simulink model "Mpc_SimMechanics_with_standing"  (R2017b)
settings: Solver=ode45  StartTime=0  StopTime=10  FixedStep=0.0005  EnableMultiTasking=on
InitFcn:
  | isSim = 1;
  | 
  | PreFunctions.CustomInitFcn_with_standing;
  | PreFunctions.simulationInitFcn_with_standing;
undefined symbols (not defined in the file): alpha_x, alpha_y, DiagnosticCodes, DynamicMatrixLibrary, motorPositions, motorVelocities, pelvisPosition, pelvisVelocity, sample_time, X, Y, Z
libraries: sm_lib x170, nesl_utility x75, Contact_Forces_Lib x6, ComponentLibrary x5, xpcrtudplib x2, slrtlib x1
(part 4 of 8)

== system Mpc_SimMechanics_with_standing/Cassie/Cassie Simulation/Cassie Pelvis ==
  Bus Element In : Inport  PortName=InBus  Element=radio
  Battery : ComponentLibrary/Simulation/Battery  SystemSampleTime=-1
  Pelvis Solid : sm_lib/Body Elements/Solid  InertiaType=Custom  Mass=10.33  MassUnits=kg  CenterOfMass=[0.05066 0.000346 0.02841]  CenterOfMassUnits=m  MomentsOfInertia=[0.085821 0.049222 0.08626]  MomentsOfInertiaUnits=kg*m^2  ProductsOfInertia=[1.276e-05 -0.00016022 -0.000414]  ProductsOfInertiaUnits=kg*m^2  DensityBased=on  Density=1000  DensityUnits=kg/(m^3)  DoExposeReferenceFrame=on  SerializedFrames=<Frames/>  GraphicType=FromGeometry  MarkerShape=Sphere  MarkerSize=10  GraphicVisPropType=SimpleVisualProperties  GraphicDiffuseColor=[0.8 0.8 0.8]  GraphicSpecularColor=[0.5 0.5 0.5 1.0]  GraphicAmbientColor=[0.5 0.5 0.5 1.0]  GraphicEmissiveColor=[0.5 0.5 0.5 1.0]  GraphicShininess=75  GraphicOpacity=1.0  GeometryShape=FromFile  RectangleSize=[1 1]  RectangleSizeUnits=m  BrickDimensions=[1 1 1]  BrickDimensionUnits=m  CylinderRadius=1  CylinderRadiusUnits=m  CylinderLength=1  CylinderLengthUnits=m  SphereRadius=1  SphereRadiusUnits=m  EllipsoidRadii=[1 1 1]  EllipsoidRadiiUnits=m  ExtrusionCrossSection=[1 1; -1 1; -1 -1; 1 -1]  ExtrusionCrossSectionUnits=m  ExtrusionLength=1  ExtrusionLengthUnits=m  PolygonNumSides=3  PolygonOuterRadius=1  PolygonOuterRadiusUnits=m  ExtGeomFileType=STL  ExtGeomFileName=cassie-pelvis.stl  ExtGeomFileUnits=m  RevolutionCrossSection=[1 1; 1 -1; 2 -1; 2 1]  RevolutionCrossSectionUnits=m  RevolutionExtent=Full  RevolutionAngle=180  RevolutionAngleUnits=deg
  Pelvis to Left Leg : sm_lib/Frames and Transforms/Rigid Transform  TranslationMethod=Cartesian  TranslationStandardOffset=0  TranslationLengthUnit=m  TranslationStandardAxis=+Z  TranslationCartesianOffset=[0.021, 0.135, 0]  TranslationROffset=0  TranslationROffsetUnits=m  TranslationZOffset=0  TranslationZOffsetUnits=m  TranslationThetaOffset=0  TranslationThetaOffsetUnits=deg  RotationMethod=RotationMatrix  RotationAngleUnits=deg  RotationStandardAxis=+Z  RotationAngle=0.0  RotationArbitraryAxis=[0 0 1]  FollAlignAxisA=+X  BaseAlignAxisA=+Y  FollAlignAxisB=+Y  BaseAlignAxisB=+Z  RotationSequenceAxes=FollowerAxes  RotationSequence=XYX  RotationSequenceAngles=[0 0 0]  RotationSequenceAnglesUnits=deg  RotationMatrix=[0, 0, 1; 0, 1, 0; -1, 0, 0]
  Pelvis to Right Leg : sm_lib/Frames and Transforms/Rigid Transform  TranslationMethod=Cartesian  TranslationStandardOffset=0  TranslationLengthUnit=m  TranslationStandardAxis=+Z  TranslationCartesianOffset=[0.021, -0.135, 0]  TranslationROffset=0  TranslationROffsetUnits=m  TranslationZOffset=0  TranslationZOffsetUnits=m  TranslationThetaOffset=0  TranslationThetaOffsetUnits=deg  RotationMethod=RotationMatrix  RotationAngleUnits=deg  RotationStandardAxis=+Z  RotationAngle=0.0  RotationArbitraryAxis=[0 0 1]  FollAlignAxisA=+X  BaseAlignAxisA=+Y  FollAlignAxisB=+Y  BaseAlignAxisB=+Z  RotationSequenceAxes=FollowerAxes  RotationSequence=XYX  RotationSequenceAngles=[0 0 0]  RotationSequenceAnglesUnits=deg  RotationMatrix=[0, 0, 1; 0, 1, 0; -1, 0, 0]
  Pelvis to VectorNav : sm_lib/Frames and Transforms/Rigid Transform  TranslationMethod=Cartesian  TranslationStandardOffset=0  TranslationLengthUnit=cm  TranslationStandardAxis=+Z  TranslationCartesianOffset=[3.155 0 -7.996]  TranslationROffset=0  TranslationROffsetUnits=m  TranslationZOffset=0  TranslationZOffsetUnits=m  TranslationThetaOffset=0  TranslationThetaOffsetUnits=deg  RotationMethod=RotationSequence  RotationAngleUnits=deg  RotationStandardAxis=+Z  RotationAngle=0.0  RotationArbitraryAxis=[0 0 1]  FollAlignAxisA=+X  BaseAlignAxisA=+Y  FollAlignAxisB=+Y  BaseAlignAxisB=+Z  RotationSequenceAxes=FollowerAxes  RotationSequence=ZYX  RotationSequenceAngles=[0 0 180]  RotationSequenceAnglesUnits=deg  RotationMatrix=[1 0 0; 0 1 0; 0 0 1]
  Radio : ComponentLibrary/Simulation/Radio  SystemSampleTime=-1
  Target PC : ComponentLibrary/Simulation/Target PC  SystemSampleTime=-1
  VectorNav : Subsystem  AncestorBlock=ComponentLibrary/Simulation/VectorNav  mask{preRotationMatrix=[1, 0, 0; 0, -1, 0; 0, 0, -1], postRotationMatrix=[1, 0, 0; 0, -1, 0; 0, 0, -1]}
      mask prompts: preRotationMatrix "Pre Rotation Matrix:"; postRotationMatrix "Post Rotation Matrix"
      mask Display: image('VectorNav.png');
  Left Leg : PMIOPort  Port=1  Side=Right
  Right Leg : PMIOPort  Port=2  Side=Right
  World : PMIOPort  Port=3  Side=Left
  Bus Element Out3 : Outport  PortName=OutBus  Element=targetPc
  Bus Element Out1 : Outport  PortName=OutBus  Element=battery
  Bus Element Out2 : Outport  PortName=OutBus  Element=radio
  Bus Element Out : Outport  PortName=OutBus  Element=vectorNav
  Bus Element Out7 : Outport  PortName=OutBus  Element=medullaCounter
  Bus Element Out8 : Outport  PortName=OutBus  Element=medullaCpuLoad
  Bus Element Out4 : Outport  PortName=OutBus  Element=bleederState
  Bus Element Out5 : Outport  PortName=OutBus  Element=leftReedSwitchState
  Bus Element Out6 : Outport  PortName=OutBus  Element=rightReedSwitchState
  Bus Element Out9 : Outport  PortName=OutBus  Element=vtmTemperature
  LinearAccelerator : Outport  Port=2
  Quaternion : Outport  Port=3
  AngularVelocity : Outport  Port=4
  IMU_pos : Outport  Port=5
  IMU_vel : Outport  Port=6
  wires:
  Target PC/1 -> Bus Element Out3/1
  Bus Element In/1 -> Radio/1
  Radio/1 -> Bus Element Out2/1
  Battery/1 -> Bus Element Out1/1
  VectorNav/1(OutBus) -> Bus Element Out/1
  VectorNav/4(AngularVelocity) -> AngularVelocity/1
  VectorNav/3(Quaternion) -> Quaternion/1
  VectorNav/2(LinearAccelerator) -> LinearAccelerator/1
  VectorNav/5(IMU_pos) -> IMU_pos/1
  VectorNav/6(IMU_vel) -> IMU_vel/1
  connections:
  Pelvis to VectorNav/RConn1 -- VectorNav/LConn1
  Pelvis to Right Leg/LConn1 -- Pelvis to VectorNav/LConn1 -- World/RConn1 -- Pelvis to Left Leg/LConn1 -- Pelvis Solid/RConn1
  Pelvis to Left Leg/RConn1 -- Left Leg/RConn1
  Pelvis to Right Leg/RConn1 -- Right Leg/RConn1
